simulink model "PID_Controller"  (R2024b)
settings: Solver=VariableStepAuto  StartTime=0.0  StopTime=20  RelTol=1e-3
model workspace (MAT data in the model file):
  Denominator = [1 -1.33793894476 0.41492381894]
  Numerator = [0 0 0.000419217442677]
libraries: slpidlib x1, simulink x1
settings Model: Creator=mafur  LastModifiedBy=mafur

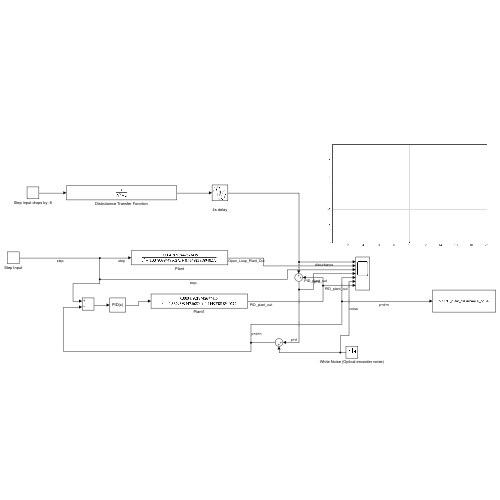
[thumbnail: Simulink's stored preview of the top-level diagram]
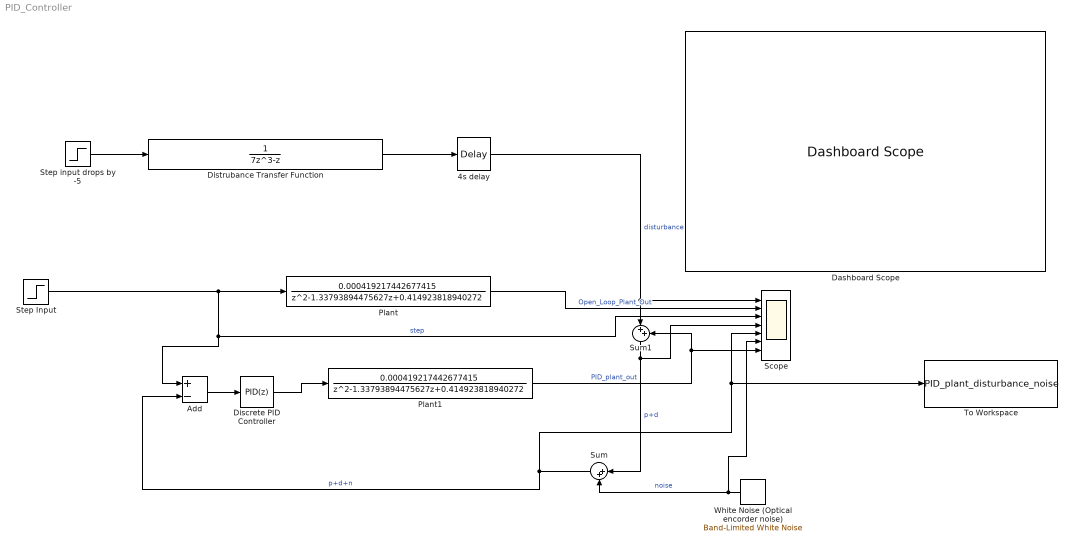
== system PID_Controller ==
  " 4s delay" : TransportDelay  DelayTime=4
  Add : Sum  Inputs=+-
  Dashboard Scope : DashboardScope
  Discrete PID Controller : slpidlib/PID Controller  Controller=PID  Form=Parallel  TimeDomain=Discrete-time  UseExternalTs=off  SampleTime=-1  IntegratorMethod=Forward Euler  FilterMethod=Forward Euler  ControllerParametersSource=internal  P=244.883045453529  I=2482.2796468479  UseKiTs=off  D=1.48430573436093  UseExternalDerivativeSource=off  N=62.3441241424031  UseFilter=on  TunerSelectOption=Transfer Function Based (PID Tuner App)  InitialConditionSource=internal  InitialConditionForIntegrator=0  InitialConditionForFilter=0  DifferentiatorICPrevScaledInput=0  ExternalReset=none  TrackingMode=off  Kt=1  LimitOutput=off  SatLimitsSource=internal  UpperSaturationLimit=inf  LowerSaturationLimit=-inf  LinearizeAsGain=off  AntiWindupMode=none  Kb=1  LimitIntegrator=off  UpperIntegratorSaturationLimit=inf  LowerIntegratorSaturationLimit=-inf  POutMin=[]  POutMax=[]  IOutMin=[]  IOutMax=[]  DOutMin=[]  DOutMax=[]  NOutMin=[]  NOutMax=[]  SumOutMin=[]  SumOutMax=[]  SaturationOutMin=[]  SaturationOutMax=[]  PParamMin=[]  PParamMax=[]  IParamMin=[]  IParamMax=[]  DParamMin=[]  DParamMax=[]  NParamMin=[]  NParamMax=[]  KbParamMin=[]  KbParamMax=[]  KtParamMin=[]  KtParamMax=[]  KbOutMin=[]  KbOutMax=[]  KtOutMin=[]  KtOutMax=[]  IntegratorOutMin=[]  IntegratorOutMax=[]  FilterOutMin=[]  FilterOutMax=[]  SumI1OutMin=[]  SumI1OutMax=[]  SumI2OutMin=[]  SumI2OutMax=[]  SumI3OutMin=[]  SumI3OutMax=[]  SumI4OutMin=[]  SumI4OutMax=[]  SumDOutMin=[]  SumDOutMax=[]  DifferentiatorOutMin=[]  DifferentiatorOutMax=[]  FilterDiffOutCoefMin=[]  FilterDiffOutCoefMax=[]  ReciprocalOutMin=[]  ReciprocalOutMax=[]  SumDenOutMin=[]  SumDenOutMax=[]  SumNumOutMin=[]  SumNumOutMax=[]  DivideOutMin=[]  DivideOutMax=[]  UdiffTsProdOutMin=[]  UdiffTsProdOutMax=[]  NTsProdOutMin=[]  NTsProdOutMax=[]  UintegralTsProdOutMin=[]  UintegralTsProdOutMax=[]  UngainTsProdOutMin=[]  UngainTsProdOutMax=[]  ClampingZeroOutDataTypeStr=Inherit: Inherit via back propagation  ClampingZeroOutMin=[]  ClampingZeroOutMax=[]  FilterDenConstantOutDataTypeStr=Inherit: Inherit via back propagation  FilterDenConstantOutMin=[]  FilterDenConstantOutMax=[]  PCopyOutDataTypeStr=Inherit: Inherit via back propagation  PCopyOutMin=[]  PCopyOutMax=[]  NCopyOutDataTypeStr=Inherit: Inherit via back propagation  NCopyOutMin=[]  NCopyOutMax=[]  IntegratorContinuousStateAttributes=''  IntegratorStateMustResolveToSignalObject=off  IntegratorRTWStateStorageClass=Auto  FilterContinuousStateAttributes=''  FilterStateMustResolveToSignalObject=off  FilterRTWStateStorageClass=Auto  ParallelPVariant=InternalParameters  IdealPVariant=Disabled  IVariant=InternalParameters  DVariant=InternalParameters  IntegratorVariant=Discrete  SatVariant=Disabled  AWVariant=Passthrough  PCopyVariant=Disabled  TRVariant=Disabled  FdbkBlocksVariant=Forward  IdealPFdbkVariant=Disabled  SatFdbkVariant=Disabled  DerivativeFilterVariant=ForwardEulerFilter  NVariant=InternalParameters  NCopyVariant=Disabled  FilterICVariant=InternalICsFilter  IntegratorICVariant=InternalICs  ExternalResetVariant=Disabled  TRSumVariant=Passthrough  SumFdbkVariant=Disabled  SumVariant=Sum_PID  TsampFilterVariant=InternalTs  TsampNgainVariant=Passthrough  TsampIntegralVariant=Disabled_SignalSpec  ExternalSaturationOutDataTypeStr=Inherit: Same as second input  DerivativeSourceVariant=ErrorSignal  PreIntVariant=InternalPreInt
      settings: LibrarySourceBlock=simulink/Discrete/Discrete PID Controller
  Distrubance Transfer Function : DiscreteTransferFcn  Denominator=[7 0 -1 0]
  Plant : DiscreteTransferFcn  Numerator=[0 0 0.000419217442677415]  Denominator=[1 -1.33793894475627 0.414923818940272]  SampleTime=0.01
  Plant1 : DiscreteTransferFcn  Numerator=[0 0 0.000419217442677415]  Denominator=[1 -1.33793894475627 0.414923818940272]  SampleTime=0.01
  Scope : Scope  NumInputPorts=7
  Step Input : Step  After=10  SampleTime=0
  Step input drops by -5 : Step  After=-5  SampleTime=0
  Sum : Sum  Inputs=|++
  Sum1 : Sum  Inputs=|++
  To Workspace : ToWorkspace  VariableName=PID_plant_disturbance_noise  SaveFormat=Structure With Time  SampleTime=-1
  White Noise (Optical encorder noise) : simulink/Sources/Band-Limited White Noise  Cov=[0.00025]  Ts=0.1  seed=[23341]
  wires:
  Plant/1 -> Scope/2  "Open_Loop_Plant_Out"
  Step Input/1 -> Add/1, Scope/3, Plant/1  "step"
  Add/1 -> Discrete PID Controller/1
  White Noise (Optical encorder noise)/1 -> Scope/6, Sum/2  "noise"
  Sum/1 -> To Workspace/1, Scope/5, Add/2  "p+d+n"
  Step input drops by -5/1 -> Distrubance Transfer Function/1
  Distrubance Transfer Function/1 -> " 4s delay"/1
  Plant1/1 -> Sum1/2, Scope/7  "PID_plant_out"
  Sum1/1 -> Sum/1, Scope/4  "p+d"
  " 4s delay"/1 -> Sum1/1, Scope/1  "disturbance"
  Discrete PID Controller/1 -> Plant1/1
